simulink model "sim_2"  (R2021b)
settings: Solver=FixedStepAuto  StartTime=0.0  StopTime=10  FixedStep=1e-3  RelTol=1e-3
values from neighbouring files (symbols this model uses):
  lambda0 = tc.lambda0_tc    [gnrt_tc.m]
  r0 = tc.r0_tc    [gnrt_tc.m]
  v_lam0 = tc.v_lam0_tc    [gnrt_tc.m]
  v_r0 = tc.v_r0_tc    [gnrt_tc.m]
  zeta = tc.zeta_tc    [gnrt_tc.m]
libraries: simulink x1
settings Model: Creator=kusha  LastModifiedBy=kusha
settings DataIOCC: SaveFormat=Array

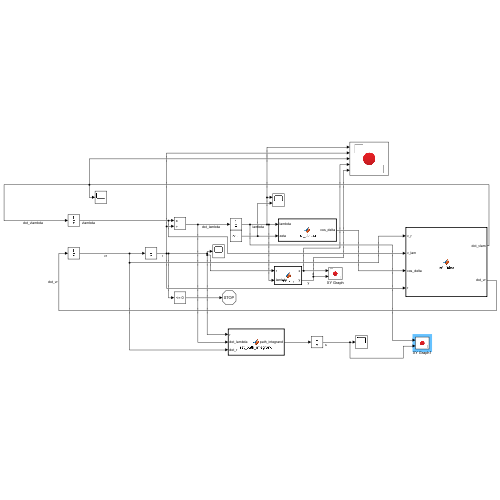
[thumbnail: Simulink's stored preview of the top-level diagram]
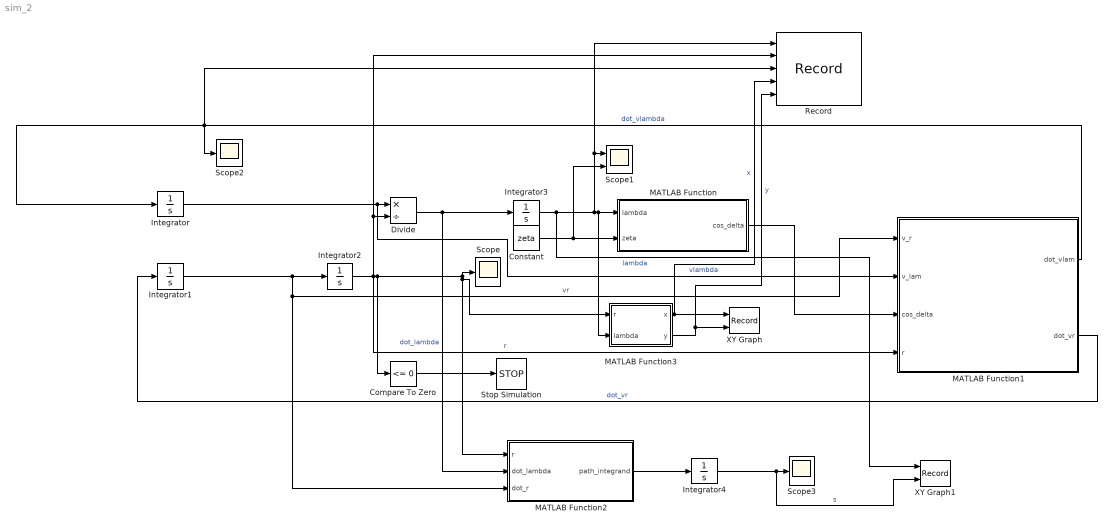
== system sim_2 ==
  Compare To Zero : simulink/Logic and Bit Operations/Compare To Zero  relop=<=  OutDataTypeStr=boolean
  Constant : Constant  Value=zeta
  Divide : Product  Inputs=*/
  Integrator : Integrator  InitialCondition=v_lam0
  Integrator1 : Integrator  InitialCondition=v_r0
  Integrator2 : Integrator  InitialCondition=r0
  Integrator3 : Integrator  InitialCondition=lambda0
  Integrator4 : Integrator  InitialCondition=lambda0
  MATLAB Function : MATLAB Function  TreatAsAtomicUnit=on
  MATLAB Function1 : MATLAB Function  TreatAsAtomicUnit=on
  MATLAB Function2 : MATLAB Function  TreatAsAtomicUnit=on
  MATLAB Function3 : MATLAB Function  TreatAsAtomicUnit=on
  Record : Record  Filename=C:\Users\kusha\Desktop\College Stuff\Year3\EE691\sim2_tc1.mat  RecordToFile=on  FileSettingsInternal="{\"entries\":[{\"content\":{\"excelSettings\":{\"content\":{},\"type\":\"Streamout.ExcelSettings\"}},\"type\":\"Streamout.FileSettingStorage\",\"uuid\":\"e284fc67-cc6b-4f24-a105-d92827d39640\"}],\"packageUris\":[\"http://schema.mathworks.com/mf0/streamout_blocks/R2020a\"],\"version\":\"1.0\"}"  Layout=[1 1]  SignalsInternal="{\"entries\":[{\"content\":{\"signals\":[{\"content\":{\"blockPath\":[\"sim_2/Record\"],\"channel\":[],\"dimensions\":[1],\"domain\":\"sim_2/Record\",\"lineColor\":\"#0072bd\",\"plots\":[1],\"port\":1,\"sid\":[\"\"],\"signalID\":6169,\"signalName\":\"lambda\"},\"type\":\"RecordBlkView.Signal\",\"uuid\":\"5e1d4593-8383-4c60-aaf1-7948e0025554\"},{\"content\":{\"blockPath\":[\"sim_2/Record\"],\"channel\":[],\"dimensions\":[1],\"domain\":\"sim_2/Record\",\"lineColor\":\"#d95319\",\"plots\":[1],\"port\":2,\"sid\":[\"\"],\"signalID\":6173,\"signalName\":\"r\"},\"type\":\"RecordBlkView.Signal\",\"uuid\":\"d0b5e290-89cf-44a9-a803-9d34fadc140e\"},{\"content\":{\"blockPath\":[\"sim_2/Record\"],\"channel\":[],\"dimensions\":[1],\"domain\":\"sim_2/Record\",\"lineColor\":\"#edb120\",\"plots\":[1],\"port\":3,\"sid\":[\"\"],\"signalID\":6177,\"signalName\":\"dot_vlambda\"},\"type\":\"RecordBlkView.Signal\",\"uuid\":\"dcc85c2b-a954-4a90-8998-d3c114ed750d\"},{\"content\":{\"blockPath\":[\"sim_2/Record\"],\"channel\":[],\"dimensions\":[1],\"domain\":\"sim_2/Record\",\"lineColor\":\"#7e2f8e\",\"plots\":[1],\"port\":4,\"sid\":[\"\"],\"signalID\":6181,\"signalName\":\"x\"},\"type\":\"RecordBlkView.Signal\",\"uuid\":\"dab1d452-d3f3-4cf7-9f1e-c7fb96d5ffdd\"},{\"content\":{\"blockPath\":[\"sim_2/Record\"],\"channel\":[],\"dimensions\":[1],\"domain\":\"sim_2/Record\",\"lineColor\":\"#77ac30\",\"plots\":[1],\"port\":5,\"sid\":[\"\"],\"signalID\":6185,\"signalName\":\"y\"},\"type\":\"RecordBlkView.Signal\",\"uuid\":\"0ce405ae-6ae6-4cb8-8434-7b237b47bb09\"}]},\"type\":\"RecordBlkView.InputSignals\",\"uuid\":\"5607a63f-f96d-4013-b166-6cf79ea52351\"}],\"packageUris\":[\"http://schema.mathworks.com/mf0/streamout_blocks/R2020a\"],\"version\":\"1.0\"}"  VisualizationBindings="{\"sparklinesplugin\":{\"info\":[{\"bindingParametersList\":[],\"subplotID\":1}]}}"
  Scope : Scope
  Scope1 : Scope  NumInputPorts=2
  Scope2 : Scope
  Scope3 : Scope
  Stop Simulation : Stop
  XY Graph : Record  FileSettingsInternal="{\"entries\":[{\"content\":{\"excelSettings\":{\"content\":{},\"type\":\"Streamout.ExcelSettings\"}},\"type\":\"Streamout.FileSettingStorage\",\"uuid\":\"cb48d0b4-73e0-4406-bdf1-c9893d5fb9ba\"}],\"packageUris\":[\"http://schema.mathworks.com/mf0/streamout_blocks/R2020a\"],\"version\":\"1.0\"}"  Layout=[1 1]  SignalsInternal="{\"entries\":[{\"content\":{\"signals\":[{\"content\":{\"blockPath\":[\"sim_2/XY Graph\"],\"channel\":[],\"dimensions\":[1],\"domain\":\"sim_2/XY Graph\",\"lineColor\":\"#4dbeee\",\"plots\":[1],\"port\":1,\"sid\":[\"\"],\"signalID\":6189,\"signalName\":\"x\"},\"type\":\"RecordBlkView.Signal\",\"uuid\":\"2721eede-f44a-4134-a284-d02dfa0021c4\"},{\"content\":{\"blockPath\":[\"sim_2/XY Graph\"],\"channel\":[],\"dimensions\":[1],\"domain\":\"sim_2/XY Graph\",\"lineColor\":\"#a2142f\",\"plots\":[1],\"port\":2,\"sid\":[\"\"],\"signalID\":6193,\"signalName\":\"y\"},\"type\":\"RecordBlkView.Signal\",\"uuid\":\"ded00bd1-f900-48f0-a299-024c3f4e4323\"}]},\"type\":\"RecordBlkView.InputSignals\",\"uuid\":\"a9aa19b4-d547-4c3f-bfc0-65a81fc06bdc\"}],\"packageUris\":[\"http://schema.mathworks.com/mf0/streamout_blocks/R2020a\"],\"version\":\"1.0\"}"  VisualizationBindings="{\"xyplotplugin\":{\"info\":[{\"series\":[{\"bindingParametersList\":[{\"parameter\":\"X-Axis\",\"signalID\":6189,\"signalName\":\"x\"},{\"parameter\":\"Y-Axis\",\"signalID\":6193,\"signalName\":\"y\"}],\"seriesID\":56134}],\"subplotID\":1}]}}"  CompatibilityTag=XY
  XY Graph1 : Record  FileSettingsInternal="{\"entries\":[{\"content\":{\"excelSettings\":{\"content\":{},\"type\":\"Streamout.ExcelSettings\"}},\"type\":\"Streamout.FileSettingStorage\",\"uuid\":\"c81034b2-02f8-4adf-b21b-cf3c38a79c28\"}],\"packageUris\":[\"http://schema.mathworks.com/mf0/streamout_blocks/R2020a\"],\"version\":\"1.0\"}"  Layout=[1 1]  SignalsInternal="{\"entries\":[{\"content\":{\"signals\":[{\"content\":{\"blockPath\":[\"sim_2/XY Graph1\"],\"channel\":[],\"dimensions\":[1],\"domain\":\"sim_2/XY Graph1\",\"lineColor\":\"#139fff\",\"plots\":[1],\"port\":1,\"sid\":[\"\"],\"signalID\":6197,\"signalName\":\"lambda\"},\"type\":\"RecordBlkView.Signal\",\"uuid\":\"1305eca3-1d9a-4038-9655-43b63bd02193\"},{\"content\":{\"blockPath\":[\"sim_2/XY Graph1\"],\"channel\":[],\"dimensions\":[1],\"domain\":\"sim_2/XY Graph1\",\"lineColor\":\"#ff6929\",\"plots\":[1],\"port\":2,\"sid\":[\"\"],\"signalID\":6201,\"signalName\":\"s\"},\"type\":\"RecordBlkView.Signal\",\"uuid\":\"c5f29761-0d63-41b6-a332-b476ce2d7013\"}]},\"type\":\"RecordBlkView.InputSignals\",\"uuid\":\"9cd7994a-cfef-45ff-8b6f-6d1f0b9f87ae\"}],\"packageUris\":[\"http://schema.mathworks.com/mf0/streamout_blocks/R2020a\"],\"version\":\"1.0\"}"  VisualizationBindings="{\"xyplotplugin\":{\"info\":[{\"series\":[{\"bindingParametersList\":[{\"parameter\":\"X-Axis\",\"signalID\":6197,\"signalName\":\"lambda\"},{\"parameter\":\"Y-Axis\",\"signalID\":6201,\"signalName\":\"s\"}],\"seriesID\":62950}],\"subplotID\":1}]}}"  CompatibilityTag=XY
  wires:
  MATLAB Function1/1(dot_vlam) -> Record/3, Integrator/1, Scope2/1  "dot_vlambda"
  Integrator/1 -> MATLAB Function1/2(v_lam), Divide/1  "vlambda"
  MATLAB Function1/2(dot_vr) -> Integrator1/1  "dot_vr"
  Integrator1/1 -> MATLAB Function1/1(v_r), MATLAB Function2/3(dot_r), Integrator2/1  "vr"
  Integrator2/1 -> Record/2, Divide/2, Compare To Zero/1, MATLAB Function3/1(r), MATLAB Function2/1(r), Scope/1, MATLAB Function1/4(r)  "r"
  Divide/1 -> Integrator3/1, MATLAB Function2/2(dot_lambda)  "dot_lambda"
  Integrator3/1 -> XY Graph1/1, Record/1, Scope1/1, MATLAB Function3/2(lambda), MATLAB Function/1(lambda)  "lambda"
  Constant/1 -> MATLAB Function/2(zeta), Scope1/2
  MATLAB Function/1(cos_delta) -> MATLAB Function1/3(cos_delta)
  MATLAB Function3/1(x) -> XY Graph/1, Record/4  "x"
  MATLAB Function3/2(y) -> XY Graph/2, Record/5  "y"
  Compare To Zero/1 -> Stop Simulation/1
  MATLAB Function2/1(path_integrand) -> Integrator4/1
  Integrator4/1 -> XY Graph1/2, Scope3/1  "s"

== matlab function sim_2/MATLAB Function1 ==
  data: v_r input; dot_vlam output; v_lam input; cos_delta input; r input; dot_vr output
function [dot_vlam, dot_vr] = ret_rates(v_r, v_lam, cos_delta, r)
dot_vlam = 2*v_r*v_lam*(cos_delta^2)/r;
dot_vr = -2*(v_lam^2)*(cos_delta^2)/r;

== matlab function sim_2/MATLAB Function ==
  data: lambda input; cos_delta output; zeta input
function cos_delta = ret_deltap(lambda, zeta)

delta = atan(2*(lambda - zeta));
cos_delta = cos(delta);

== matlab function sim_2/MATLAB Function2 ==
  data: r input; path_integrand output; dot_lambda input; dot_r input
function path_integrand = ret_path_integrand(r, dot_lambda, dot_r)

path_integrand = sqrt(r^2 + (dot_r/dot_lambda)^2)*abs(dot_lambda);

== matlab function sim_2/MATLAB Function3 ==
  data: x output; r input; y output; lambda input
function [x, y] = ret_x_y(r, lambda)

x = r*cos(lambda);
y = r*sin(lambda);
